simulink model "rx2"  (R2022b)
settings: Solver=FixedStepDiscrete  StartTime=0.0  StopTime=3.3E6  FixedStep=1  RelTol=1e-3  EnableMultiTasking=on
model workspace (MAT data in the model file):
  mwTaskManagerKernelLatency = 0
undefined symbols (not defined in the file or in its folder): Add, jsin, magnitude, rom_pilot_conj_tt, Shift
libraries: hdlsllib x3231, whdlutilities x525, simulink x260, whdlmod x112, whdledac x26, dsphdlmathfun2 x24, commchan3 x1
(part 5 of 59)

== system rx2/process divide/transport_block3/Subsystem8 ==
  data_in : Inport
  select_valid : Inport  Port=2  OutDataTypeStr=boolean
  Constant : Constant  Value=0  OutDataTypeStr=fixdt(1,16,14)
  Real-Imag to Complex : RealImagToComplex
  Switch : Switch  Criteria=u2 ~= 0  SaturateOnIntegerOverflow=off  InputSameDT=off
  ctrl_gen : Subsystem
  data_out : Outport
  ctrl_out : Outport  Port=2
  wires:
  Real-Imag to Complex/1 -> Switch/3
  data_in/1 -> Switch/1
  ctrl_gen/2(ctrl_out) -> ctrl_out/1
  ctrl_gen/1(data_out) -> data_out/1
  select_valid/1 -> Switch/2, ctrl_gen/2(valid_in)
  Constant/1 -> Real-Imag to Complex/1, Real-Imag to Complex/2
  Switch/1 -> ctrl_gen/1(data_in)

== system rx2/process divide/transport_block3/Subsystem9 ==
  data_in : Inport
  select_valid : Inport  Port=2  OutDataTypeStr=boolean
  Constant : Constant  Value=0  OutDataTypeStr=fixdt(1,16,14)
  Real-Imag to Complex : RealImagToComplex
  Switch : Switch  Criteria=u2 ~= 0  SaturateOnIntegerOverflow=off  InputSameDT=off
  ctrl_gen : Subsystem
  data_out : Outport
  ctrl_out : Outport  Port=2
  wires:
  Real-Imag to Complex/1 -> Switch/3
  data_in/1 -> Switch/1
  ctrl_gen/2(ctrl_out) -> ctrl_out/1
  ctrl_gen/1(data_out) -> data_out/1
  select_valid/1 -> Switch/2, ctrl_gen/2(valid_in)
  Constant/1 -> Real-Imag to Complex/1, Real-Imag to Complex/2
  Switch/1 -> ctrl_gen/1(data_in)

== system rx2/process divide/transport_block4/Subsystem1 ==
  data_in : Inport
  select_valid : Inport  Port=2  OutDataTypeStr=boolean
  Constant : Constant  Value=0  OutDataTypeStr=fixdt(1,16,14)
  Real-Imag to Complex : RealImagToComplex
  Switch : Switch  Criteria=u2 ~= 0  SaturateOnIntegerOverflow=off  InputSameDT=off
  ctrl_gen : Subsystem
  data_out : Outport
  ctrl_out : Outport  Port=2
  wires:
  Real-Imag to Complex/1 -> Switch/3
  data_in/1 -> Switch/1
  ctrl_gen/2(ctrl_out) -> ctrl_out/1
  ctrl_gen/1(data_out) -> data_out/1
  select_valid/1 -> Switch/2, ctrl_gen/2(valid_in)
  Constant/1 -> Real-Imag to Complex/1, Real-Imag to Complex/2
  Switch/1 -> ctrl_gen/1(data_in)

== system rx2/process divide/transport_block4/Subsystem10 ==
  data_in : Inport
  select_valid : Inport  Port=2  OutDataTypeStr=boolean
  Constant : Constant  Value=0  OutDataTypeStr=fixdt(1,16,14)
  Real-Imag to Complex : RealImagToComplex
  Switch : Switch  Criteria=u2 ~= 0  SaturateOnIntegerOverflow=off  InputSameDT=off
  ctrl_gen : Subsystem
  data_out : Outport
  ctrl_out : Outport  Port=2
  wires:
  Switch/1 -> ctrl_gen/1(data_in)
  Constant/1 -> Real-Imag to Complex/2, Real-Imag to Complex/1
  select_valid/1 -> ctrl_gen/2(valid_in), Switch/2
  ctrl_gen/1(data_out) -> data_out/1
  ctrl_gen/2(ctrl_out) -> ctrl_out/1
  data_in/1 -> Switch/1
  Real-Imag to Complex/1 -> Switch/3

== system rx2/process divide/transport_block4/Subsystem11 ==
  data_in : Inport
  select_valid : Inport  Port=2  OutDataTypeStr=boolean
  Constant : Constant  Value=0  OutDataTypeStr=fixdt(1,16,14)
  Real-Imag to Complex : RealImagToComplex
  Switch : Switch  Criteria=u2 ~= 0  SaturateOnIntegerOverflow=off  InputSameDT=off
  ctrl_gen : Subsystem
  data_out : Outport
  ctrl_out : Outport  Port=2
  wires:
  Switch/1 -> ctrl_gen/1(data_in)
  Constant/1 -> Real-Imag to Complex/2, Real-Imag to Complex/1
  select_valid/1 -> ctrl_gen/2(valid_in), Switch/2
  ctrl_gen/1(data_out) -> data_out/1
  ctrl_gen/2(ctrl_out) -> ctrl_out/1
  data_in/1 -> Switch/1
  Real-Imag to Complex/1 -> Switch/3

== system rx2/process divide/transport_block4/Subsystem12 ==
  data_in : Inport
  select_valid : Inport  Port=2  OutDataTypeStr=boolean
  Constant : Constant  Value=0  OutDataTypeStr=fixdt(1,16,14)
  Real-Imag to Complex : RealImagToComplex
  Switch : Switch  Criteria=u2 ~= 0  SaturateOnIntegerOverflow=off  InputSameDT=off
  ctrl_gen : Subsystem
  data_out : Outport
  ctrl_out : Outport  Port=2
  wires:
  Switch/1 -> ctrl_gen/1(data_in)
  Constant/1 -> Real-Imag to Complex/2, Real-Imag to Complex/1
  select_valid/1 -> ctrl_gen/2(valid_in), Switch/2
  ctrl_gen/1(data_out) -> data_out/1
  ctrl_gen/2(ctrl_out) -> ctrl_out/1
  data_in/1 -> Switch/1
  Real-Imag to Complex/1 -> Switch/3

== system rx2/process divide/transport_block4/Subsystem13 ==
  data_in : Inport
  select_valid : Inport  Port=2  OutDataTypeStr=boolean
  Constant : Constant  Value=0  OutDataTypeStr=fixdt(1,16,14)
  Real-Imag to Complex : RealImagToComplex
  Switch : Switch  Criteria=u2 ~= 0  SaturateOnIntegerOverflow=off  InputSameDT=off
  ctrl_gen : Subsystem
  data_out : Outport
  ctrl_out : Outport  Port=2
  wires:
  Switch/1 -> ctrl_gen/1(data_in)
  Constant/1 -> Real-Imag to Complex/2, Real-Imag to Complex/1
  select_valid/1 -> ctrl_gen/2(valid_in), Switch/2
  ctrl_gen/1(data_out) -> data_out/1
  ctrl_gen/2(ctrl_out) -> ctrl_out/1
  data_in/1 -> Switch/1
  Real-Imag to Complex/1 -> Switch/3

== system rx2/process divide/transport_block4/Subsystem14 ==
  data_in : Inport
  select_valid : Inport  Port=2  OutDataTypeStr=boolean
  Constant : Constant  Value=0  OutDataTypeStr=fixdt(1,16,14)
  Real-Imag to Complex : RealImagToComplex
  Switch : Switch  Criteria=u2 ~= 0  SaturateOnIntegerOverflow=off  InputSameDT=off
  ctrl_gen : Subsystem
  data_out : Outport
  ctrl_out : Outport  Port=2
  wires:
  Switch/1 -> ctrl_gen/1(data_in)
  Constant/1 -> Real-Imag to Complex/2, Real-Imag to Complex/1
  select_valid/1 -> ctrl_gen/2(valid_in), Switch/2
  ctrl_gen/1(data_out) -> data_out/1
  ctrl_gen/2(ctrl_out) -> ctrl_out/1
  data_in/1 -> Switch/1
  Real-Imag to Complex/1 -> Switch/3

== system rx2/process divide/transport_block4/Subsystem2 ==
  data_in : Inport
  select_valid : Inport  Port=2  OutDataTypeStr=boolean
  Constant : Constant  Value=0  OutDataTypeStr=fixdt(1,16,14)
  Real-Imag to Complex : RealImagToComplex
  Switch : Switch  Criteria=u2 ~= 0  SaturateOnIntegerOverflow=off  InputSameDT=off
  ctrl_gen : Subsystem
  data_out : Outport
  ctrl_out : Outport  Port=2
  wires:
  Switch/1 -> ctrl_gen/1(data_in)
  Constant/1 -> Real-Imag to Complex/2, Real-Imag to Complex/1
  select_valid/1 -> ctrl_gen/2(valid_in), Switch/2
  ctrl_gen/1(data_out) -> data_out/1
  ctrl_gen/2(ctrl_out) -> ctrl_out/1
  data_in/1 -> Switch/1
  Real-Imag to Complex/1 -> Switch/3

== system rx2/process divide/transport_block4/Subsystem3 ==
  data_in : Inport
  select_valid : Inport  Port=2  OutDataTypeStr=boolean
  Constant : Constant  Value=0  OutDataTypeStr=fixdt(1,16,14)
  Real-Imag to Complex : RealImagToComplex
  Switch : Switch  Criteria=u2 ~= 0  SaturateOnIntegerOverflow=off  InputSameDT=off
  ctrl_gen : Subsystem
  data_out : Outport
  ctrl_out : Outport  Port=2
  wires:
  Real-Imag to Complex/1 -> Switch/3
  data_in/1 -> Switch/1
  ctrl_gen/2(ctrl_out) -> ctrl_out/1
  ctrl_gen/1(data_out) -> data_out/1
  select_valid/1 -> Switch/2, ctrl_gen/2(valid_in)
  Constant/1 -> Real-Imag to Complex/1, Real-Imag to Complex/2
  Switch/1 -> ctrl_gen/1(data_in)

== system rx2/process divide/transport_block4/Subsystem4 ==
  data_in : Inport
  select_valid : Inport  Port=2  OutDataTypeStr=boolean
  Constant : Constant  Value=0  OutDataTypeStr=fixdt(1,16,14)
  Real-Imag to Complex : RealImagToComplex
  Switch : Switch  Criteria=u2 ~= 0  SaturateOnIntegerOverflow=off  InputSameDT=off
  ctrl_gen : Subsystem
  data_out : Outport
  ctrl_out : Outport  Port=2
  wires:
  Switch/1 -> ctrl_gen/1(data_in)
  Constant/1 -> Real-Imag to Complex/2, Real-Imag to Complex/1
  select_valid/1 -> ctrl_gen/2(valid_in), Switch/2
  ctrl_gen/1(data_out) -> data_out/1
  ctrl_gen/2(ctrl_out) -> ctrl_out/1
  data_in/1 -> Switch/1
  Real-Imag to Complex/1 -> Switch/3

== system rx2/process divide/transport_block4/Subsystem5 ==
  data_in : Inport
  select_valid : Inport  Port=2  OutDataTypeStr=boolean
  Constant : Constant  Value=0  OutDataTypeStr=fixdt(1,16,14)
  Real-Imag to Complex : RealImagToComplex
  Switch : Switch  Criteria=u2 ~= 0  SaturateOnIntegerOverflow=off  InputSameDT=off
  ctrl_gen : Subsystem
  data_out : Outport
  ctrl_out : Outport  Port=2
  wires:
  Switch/1 -> ctrl_gen/1(data_in)
  Constant/1 -> Real-Imag to Complex/2, Real-Imag to Complex/1
  select_valid/1 -> ctrl_gen/2(valid_in), Switch/2
  ctrl_gen/1(data_out) -> data_out/1
  ctrl_gen/2(ctrl_out) -> ctrl_out/1
  data_in/1 -> Switch/1
  Real-Imag to Complex/1 -> Switch/3

== system rx2/process divide/transport_block4/Subsystem6 ==
  data_in : Inport
  select_valid : Inport  Port=2  OutDataTypeStr=boolean
  Constant : Constant  Value=0  OutDataTypeStr=fixdt(1,16,14)
  Real-Imag to Complex : RealImagToComplex
  Switch : Switch  Criteria=u2 ~= 0  SaturateOnIntegerOverflow=off  InputSameDT=off
  ctrl_gen : Subsystem
  data_out : Outport
  ctrl_out : Outport  Port=2
  wires:
  Switch/1 -> ctrl_gen/1(data_in)
  Constant/1 -> Real-Imag to Complex/2, Real-Imag to Complex/1
  select_valid/1 -> ctrl_gen/2(valid_in), Switch/2
  ctrl_gen/1(data_out) -> data_out/1
  ctrl_gen/2(ctrl_out) -> ctrl_out/1
  data_in/1 -> Switch/1
  Real-Imag to Complex/1 -> Switch/3

== system rx2/process divide/transport_block4/Subsystem7 ==
  data_in : Inport
  select_valid : Inport  Port=2  OutDataTypeStr=boolean
  Constant : Constant  Value=0  OutDataTypeStr=fixdt(1,16,14)
  Real-Imag to Complex : RealImagToComplex
  Switch : Switch  Criteria=u2 ~= 0  SaturateOnIntegerOverflow=off  InputSameDT=off
  ctrl_gen : Subsystem
  data_out : Outport
  ctrl_out : Outport  Port=2
  wires:
  Switch/1 -> ctrl_gen/1(data_in)
  Constant/1 -> Real-Imag to Complex/2, Real-Imag to Complex/1
  select_valid/1 -> ctrl_gen/2(valid_in), Switch/2
  ctrl_gen/1(data_out) -> data_out/1
  ctrl_gen/2(ctrl_out) -> ctrl_out/1
  data_in/1 -> Switch/1
  Real-Imag to Complex/1 -> Switch/3

== system rx2/process divide/transport_block4/Subsystem8 ==
  data_in : Inport
  select_valid : Inport  Port=2  OutDataTypeStr=boolean
  Constant : Constant  Value=0  OutDataTypeStr=fixdt(1,16,14)
  Real-Imag to Complex : RealImagToComplex
  Switch : Switch  Criteria=u2 ~= 0  SaturateOnIntegerOverflow=off  InputSameDT=off
  ctrl_gen : Subsystem
  data_out : Outport
  ctrl_out : Outport  Port=2
  wires:
  Switch/1 -> ctrl_gen/1(data_in)
  Constant/1 -> Real-Imag to Complex/2, Real-Imag to Complex/1
  select_valid/1 -> ctrl_gen/2(valid_in), Switch/2
  ctrl_gen/1(data_out) -> data_out/1
  ctrl_gen/2(ctrl_out) -> ctrl_out/1
  data_in/1 -> Switch/1
  Real-Imag to Complex/1 -> Switch/3

== system rx2/process divide/transport_block4/Subsystem9 ==
  data_in : Inport
  select_valid : Inport  Port=2  OutDataTypeStr=boolean
  Constant : Constant  Value=0  OutDataTypeStr=fixdt(1,16,14)
  Real-Imag to Complex : RealImagToComplex
  Switch : Switch  Criteria=u2 ~= 0  SaturateOnIntegerOverflow=off  InputSameDT=off
  ctrl_gen : Subsystem
  data_out : Outport
  ctrl_out : Outport  Port=2
  wires:
  Switch/1 -> ctrl_gen/1(data_in)
  Constant/1 -> Real-Imag to Complex/2, Real-Imag to Complex/1
  select_valid/1 -> ctrl_gen/2(valid_in), Switch/2
  ctrl_gen/1(data_out) -> data_out/1
  ctrl_gen/2(ctrl_out) -> ctrl_out/1
  data_in/1 -> Switch/1
  Real-Imag to Complex/1 -> Switch/3

== system rx2/process divide/transport_block5/Subsystem1 ==
  data_in : Inport
  select_valid : Inport  Port=2  OutDataTypeStr=boolean
  Constant : Constant  Value=0  OutDataTypeStr=fixdt(1,16,14)
  Real-Imag to Complex : RealImagToComplex
  Switch : Switch  Criteria=u2 ~= 0  SaturateOnIntegerOverflow=off  InputSameDT=off
  ctrl_gen : Subsystem
  data_out : Outport
  ctrl_out : Outport  Port=2
  wires:
  Switch/1 -> ctrl_gen/1(data_in)
  Constant/1 -> Real-Imag to Complex/2, Real-Imag to Complex/1
  select_valid/1 -> ctrl_gen/2(valid_in), Switch/2
  ctrl_gen/1(data_out) -> data_out/1
  ctrl_gen/2(ctrl_out) -> ctrl_out/1
  data_in/1 -> Switch/1
  Real-Imag to Complex/1 -> Switch/3

== system rx2/process divide/transport_block5/Subsystem10 ==
  data_in : Inport
  select_valid : Inport  Port=2  OutDataTypeStr=boolean
  Constant : Constant  Value=0  OutDataTypeStr=fixdt(1,16,14)
  Real-Imag to Complex : RealImagToComplex
  Switch : Switch  Criteria=u2 ~= 0  SaturateOnIntegerOverflow=off  InputSameDT=off
  ctrl_gen : Subsystem
  data_out : Outport
  ctrl_out : Outport  Port=2
  wires:
  Real-Imag to Complex/1 -> Switch/3
  data_in/1 -> Switch/1
  ctrl_gen/2(ctrl_out) -> ctrl_out/1
  ctrl_gen/1(data_out) -> data_out/1
  select_valid/1 -> Switch/2, ctrl_gen/2(valid_in)
  Constant/1 -> Real-Imag to Complex/1, Real-Imag to Complex/2
  Switch/1 -> ctrl_gen/1(data_in)

== system rx2/process divide/transport_block5/Subsystem11 ==
  data_in : Inport
  select_valid : Inport  Port=2  OutDataTypeStr=boolean
  Constant : Constant  Value=0  OutDataTypeStr=fixdt(1,16,14)
  Real-Imag to Complex : RealImagToComplex
  Switch : Switch  Criteria=u2 ~= 0  SaturateOnIntegerOverflow=off  InputSameDT=off
  ctrl_gen : Subsystem
  data_out : Outport
  ctrl_out : Outport  Port=2
  wires:
  Real-Imag to Complex/1 -> Switch/3
  data_in/1 -> Switch/1
  ctrl_gen/2(ctrl_out) -> ctrl_out/1
  ctrl_gen/1(data_out) -> data_out/1
  select_valid/1 -> Switch/2, ctrl_gen/2(valid_in)
  Constant/1 -> Real-Imag to Complex/1, Real-Imag to Complex/2
  Switch/1 -> ctrl_gen/1(data_in)

== system rx2/process divide/transport_block5/Subsystem12 ==
  data_in : Inport
  select_valid : Inport  Port=2  OutDataTypeStr=boolean
  Constant : Constant  Value=0  OutDataTypeStr=fixdt(1,16,14)
  Real-Imag to Complex : RealImagToComplex
  Switch : Switch  Criteria=u2 ~= 0  SaturateOnIntegerOverflow=off  InputSameDT=off
  ctrl_gen : Subsystem
  data_out : Outport
  ctrl_out : Outport  Port=2
  wires:
  Real-Imag to Complex/1 -> Switch/3
  data_in/1 -> Switch/1
  ctrl_gen/2(ctrl_out) -> ctrl_out/1
  ctrl_gen/1(data_out) -> data_out/1
  select_valid/1 -> Switch/2, ctrl_gen/2(valid_in)
  Constant/1 -> Real-Imag to Complex/1, Real-Imag to Complex/2
  Switch/1 -> ctrl_gen/1(data_in)

== system rx2/process divide/transport_block5/Subsystem13 ==
  data_in : Inport
  select_valid : Inport  Port=2  OutDataTypeStr=boolean
  Constant : Constant  Value=0  OutDataTypeStr=fixdt(1,16,14)
  Real-Imag to Complex : RealImagToComplex
  Switch : Switch  Criteria=u2 ~= 0  SaturateOnIntegerOverflow=off  InputSameDT=off
  ctrl_gen : Subsystem
  data_out : Outport
  ctrl_out : Outport  Port=2
  wires:
  Real-Imag to Complex/1 -> Switch/3
  data_in/1 -> Switch/1
  ctrl_gen/2(ctrl_out) -> ctrl_out/1
  ctrl_gen/1(data_out) -> data_out/1
  select_valid/1 -> Switch/2, ctrl_gen/2(valid_in)
  Constant/1 -> Real-Imag to Complex/1, Real-Imag to Complex/2
  Switch/1 -> ctrl_gen/1(data_in)

== system rx2/process divide/transport_block5/Subsystem14 ==
  data_in : Inport
  select_valid : Inport  Port=2  OutDataTypeStr=boolean
  Constant : Constant  Value=0  OutDataTypeStr=fixdt(1,16,14)
  Real-Imag to Complex : RealImagToComplex
  Switch : Switch  Criteria=u2 ~= 0  SaturateOnIntegerOverflow=off  InputSameDT=off
  ctrl_gen : Subsystem
  data_out : Outport
  ctrl_out : Outport  Port=2
  wires:
  Real-Imag to Complex/1 -> Switch/3
  data_in/1 -> Switch/1
  ctrl_gen/2(ctrl_out) -> ctrl_out/1
  ctrl_gen/1(data_out) -> data_out/1
  select_valid/1 -> Switch/2, ctrl_gen/2(valid_in)
  Constant/1 -> Real-Imag to Complex/1, Real-Imag to Complex/2
  Switch/1 -> ctrl_gen/1(data_in)

== system rx2/process divide/transport_block5/Subsystem2 ==
  data_in : Inport
  select_valid : Inport  Port=2  OutDataTypeStr=boolean
  Constant : Constant  Value=0  OutDataTypeStr=fixdt(1,16,14)
  Real-Imag to Complex : RealImagToComplex
  Switch : Switch  Criteria=u2 ~= 0  SaturateOnIntegerOverflow=off  InputSameDT=off
  ctrl_gen : Subsystem
  data_out : Outport
  ctrl_out : Outport  Port=2
  wires:
  Real-Imag to Complex/1 -> Switch/3
  data_in/1 -> Switch/1
  ctrl_gen/2(ctrl_out) -> ctrl_out/1
  ctrl_gen/1(data_out) -> data_out/1
  select_valid/1 -> Switch/2, ctrl_gen/2(valid_in)
  Constant/1 -> Real-Imag to Complex/1, Real-Imag to Complex/2
  Switch/1 -> ctrl_gen/1(data_in)

== system rx2/process divide/transport_block5/Subsystem3 ==
  data_in : Inport
  select_valid : Inport  Port=2  OutDataTypeStr=boolean
  Constant : Constant  Value=0  OutDataTypeStr=fixdt(1,16,14)
  Real-Imag to Complex : RealImagToComplex
  Switch : Switch  Criteria=u2 ~= 0  SaturateOnIntegerOverflow=off  InputSameDT=off
  ctrl_gen : Subsystem
  data_out : Outport
  ctrl_out : Outport  Port=2
  wires:
  Switch/1 -> ctrl_gen/1(data_in)
  Constant/1 -> Real-Imag to Complex/2, Real-Imag to Complex/1
  select_valid/1 -> ctrl_gen/2(valid_in), Switch/2
  ctrl_gen/1(data_out) -> data_out/1
  ctrl_gen/2(ctrl_out) -> ctrl_out/1
  data_in/1 -> Switch/1
  Real-Imag to Complex/1 -> Switch/3

== system rx2/process divide/transport_block5/Subsystem4 ==
  data_in : Inport
  select_valid : Inport  Port=2  OutDataTypeStr=boolean
  Constant : Constant  Value=0  OutDataTypeStr=fixdt(1,16,14)
  Real-Imag to Complex : RealImagToComplex
  Switch : Switch  Criteria=u2 ~= 0  SaturateOnIntegerOverflow=off  InputSameDT=off
  ctrl_gen : Subsystem
  data_out : Outport
  ctrl_out : Outport  Port=2
  wires:
  Real-Imag to Complex/1 -> Switch/3
  data_in/1 -> Switch/1
  ctrl_gen/2(ctrl_out) -> ctrl_out/1
  ctrl_gen/1(data_out) -> data_out/1
  select_valid/1 -> Switch/2, ctrl_gen/2(valid_in)
  Constant/1 -> Real-Imag to Complex/1, Real-Imag to Complex/2
  Switch/1 -> ctrl_gen/1(data_in)

== system rx2/process divide/transport_block5/Subsystem5 ==
  data_in : Inport
  select_valid : Inport  Port=2  OutDataTypeStr=boolean
  Constant : Constant  Value=0  OutDataTypeStr=fixdt(1,16,14)
  Real-Imag to Complex : RealImagToComplex
  Switch : Switch  Criteria=u2 ~= 0  SaturateOnIntegerOverflow=off  InputSameDT=off
  ctrl_gen : Subsystem
  data_out : Outport
  ctrl_out : Outport  Port=2
  wires:
  Real-Imag to Complex/1 -> Switch/3
  data_in/1 -> Switch/1
  ctrl_gen/2(ctrl_out) -> ctrl_out/1
  ctrl_gen/1(data_out) -> data_out/1
  select_valid/1 -> Switch/2, ctrl_gen/2(valid_in)
  Constant/1 -> Real-Imag to Complex/1, Real-Imag to Complex/2
  Switch/1 -> ctrl_gen/1(data_in)

== system rx2/process divide/transport_block5/Subsystem6 ==
  data_in : Inport
  select_valid : Inport  Port=2  OutDataTypeStr=boolean
  Constant : Constant  Value=0  OutDataTypeStr=fixdt(1,16,14)
  Real-Imag to Complex : RealImagToComplex
  Switch : Switch  Criteria=u2 ~= 0  SaturateOnIntegerOverflow=off  InputSameDT=off
  ctrl_gen : Subsystem
  data_out : Outport
  ctrl_out : Outport  Port=2
  wires:
  Real-Imag to Complex/1 -> Switch/3
  data_in/1 -> Switch/1
  ctrl_gen/2(ctrl_out) -> ctrl_out/1
  ctrl_gen/1(data_out) -> data_out/1
  select_valid/1 -> Switch/2, ctrl_gen/2(valid_in)
  Constant/1 -> Real-Imag to Complex/1, Real-Imag to Complex/2
  Switch/1 -> ctrl_gen/1(data_in)

== system rx2/process divide/transport_block5/Subsystem7 ==
  data_in : Inport
  select_valid : Inport  Port=2  OutDataTypeStr=boolean
  Constant : Constant  Value=0  OutDataTypeStr=fixdt(1,16,14)
  Real-Imag to Complex : RealImagToComplex
  Switch : Switch  Criteria=u2 ~= 0  SaturateOnIntegerOverflow=off  InputSameDT=off
  ctrl_gen : Subsystem
  data_out : Outport
  ctrl_out : Outport  Port=2
  wires:
  Real-Imag to Complex/1 -> Switch/3
  data_in/1 -> Switch/1
  ctrl_gen/2(ctrl_out) -> ctrl_out/1
  ctrl_gen/1(data_out) -> data_out/1
  select_valid/1 -> Switch/2, ctrl_gen/2(valid_in)
  Constant/1 -> Real-Imag to Complex/1, Real-Imag to Complex/2
  Switch/1 -> ctrl_gen/1(data_in)

== system rx2/process divide/transport_block5/Subsystem8 ==
  data_in : Inport
  select_valid : Inport  Port=2  OutDataTypeStr=boolean
  Constant : Constant  Value=0  OutDataTypeStr=fixdt(1,16,14)
  Real-Imag to Complex : RealImagToComplex
  Switch : Switch  Criteria=u2 ~= 0  SaturateOnIntegerOverflow=off  InputSameDT=off
  ctrl_gen : Subsystem
  data_out : Outport
  ctrl_out : Outport  Port=2
  wires:
  Real-Imag to Complex/1 -> Switch/3
  data_in/1 -> Switch/1
  ctrl_gen/2(ctrl_out) -> ctrl_out/1
  ctrl_gen/1(data_out) -> data_out/1
  select_valid/1 -> Switch/2, ctrl_gen/2(valid_in)
  Constant/1 -> Real-Imag to Complex/1, Real-Imag to Complex/2
  Switch/1 -> ctrl_gen/1(data_in)

== system rx2/process divide/transport_block5/Subsystem9 ==
  data_in : Inport
  select_valid : Inport  Port=2  OutDataTypeStr=boolean
  Constant : Constant  Value=0  OutDataTypeStr=fixdt(1,16,14)
  Real-Imag to Complex : RealImagToComplex
  Switch : Switch  Criteria=u2 ~= 0  SaturateOnIntegerOverflow=off  InputSameDT=off
  ctrl_gen : Subsystem
  data_out : Outport
  ctrl_out : Outport  Port=2
  wires:
  Real-Imag to Complex/1 -> Switch/3
  data_in/1 -> Switch/1
  ctrl_gen/2(ctrl_out) -> ctrl_out/1
  ctrl_gen/1(data_out) -> data_out/1
  select_valid/1 -> Switch/2, ctrl_gen/2(valid_in)
  Constant/1 -> Real-Imag to Complex/1, Real-Imag to Complex/2
  Switch/1 -> ctrl_gen/1(data_in)

== system rx2/process divide/transport_block6/Subsystem1 ==
  data_in : Inport
  select_valid : Inport  Port=2  OutDataTypeStr=boolean
  Constant : Constant  Value=0  OutDataTypeStr=fixdt(1,16,14)
  Real-Imag to Complex : RealImagToComplex
  Switch : Switch  Criteria=u2 ~= 0  SaturateOnIntegerOverflow=off  InputSameDT=off
  ctrl_gen : Subsystem
  data_out : Outport
  ctrl_out : Outport  Port=2
  wires:
  Real-Imag to Complex/1 -> Switch/3
  data_in/1 -> Switch/1
  ctrl_gen/2(ctrl_out) -> ctrl_out/1
  ctrl_gen/1(data_out) -> data_out/1
  select_valid/1 -> Switch/2, ctrl_gen/2(valid_in)
  Constant/1 -> Real-Imag to Complex/1, Real-Imag to Complex/2
  Switch/1 -> ctrl_gen/1(data_in)

== system rx2/process divide/transport_block6/Subsystem10 ==
  data_in : Inport
  select_valid : Inport  Port=2  OutDataTypeStr=boolean
  Constant : Constant  Value=0  OutDataTypeStr=fixdt(1,16,14)
  Real-Imag to Complex : RealImagToComplex
  Switch : Switch  Criteria=u2 ~= 0  SaturateOnIntegerOverflow=off  InputSameDT=off
  ctrl_gen : Subsystem
  data_out : Outport
  ctrl_out : Outport  Port=2
  wires:
  Switch/1 -> ctrl_gen/1(data_in)
  Constant/1 -> Real-Imag to Complex/2, Real-Imag to Complex/1
  select_valid/1 -> ctrl_gen/2(valid_in), Switch/2
  ctrl_gen/1(data_out) -> data_out/1
  ctrl_gen/2(ctrl_out) -> ctrl_out/1
  data_in/1 -> Switch/1
  Real-Imag to Complex/1 -> Switch/3

== system rx2/process divide/transport_block6/Subsystem11 ==
  data_in : Inport
  select_valid : Inport  Port=2  OutDataTypeStr=boolean
  Constant : Constant  Value=0  OutDataTypeStr=fixdt(1,16,14)
  Real-Imag to Complex : RealImagToComplex
  Switch : Switch  Criteria=u2 ~= 0  SaturateOnIntegerOverflow=off  InputSameDT=off
  ctrl_gen : Subsystem
  data_out : Outport
  ctrl_out : Outport  Port=2
  wires:
  Switch/1 -> ctrl_gen/1(data_in)
  Constant/1 -> Real-Imag to Complex/2, Real-Imag to Complex/1
  select_valid/1 -> ctrl_gen/2(valid_in), Switch/2
  ctrl_gen/1(data_out) -> data_out/1
  ctrl_gen/2(ctrl_out) -> ctrl_out/1
  data_in/1 -> Switch/1
  Real-Imag to Complex/1 -> Switch/3

== system rx2/process divide/transport_block6/Subsystem12 ==
  data_in : Inport
  select_valid : Inport  Port=2  OutDataTypeStr=boolean
  Constant : Constant  Value=0  OutDataTypeStr=fixdt(1,16,14)
  Real-Imag to Complex : RealImagToComplex
  Switch : Switch  Criteria=u2 ~= 0  SaturateOnIntegerOverflow=off  InputSameDT=off
  ctrl_gen : Subsystem
  data_out : Outport
  ctrl_out : Outport  Port=2
  wires:
  Switch/1 -> ctrl_gen/1(data_in)
  Constant/1 -> Real-Imag to Complex/2, Real-Imag to Complex/1
  select_valid/1 -> ctrl_gen/2(valid_in), Switch/2
  ctrl_gen/1(data_out) -> data_out/1
  ctrl_gen/2(ctrl_out) -> ctrl_out/1
  data_in/1 -> Switch/1
  Real-Imag to Complex/1 -> Switch/3

== system rx2/process divide/transport_block6/Subsystem13 ==
  data_in : Inport
  select_valid : Inport  Port=2  OutDataTypeStr=boolean
  Constant : Constant  Value=0  OutDataTypeStr=fixdt(1,16,14)
  Real-Imag to Complex : RealImagToComplex
  Switch : Switch  Criteria=u2 ~= 0  SaturateOnIntegerOverflow=off  InputSameDT=off
  ctrl_gen : Subsystem
  data_out : Outport
  ctrl_out : Outport  Port=2
  wires:
  Switch/1 -> ctrl_gen/1(data_in)
  Constant/1 -> Real-Imag to Complex/2, Real-Imag to Complex/1
  select_valid/1 -> ctrl_gen/2(valid_in), Switch/2
  ctrl_gen/1(data_out) -> data_out/1
  ctrl_gen/2(ctrl_out) -> ctrl_out/1
  data_in/1 -> Switch/1
  Real-Imag to Complex/1 -> Switch/3

== system rx2/process divide/transport_block6/Subsystem14 ==
  data_in : Inport
  select_valid : Inport  Port=2  OutDataTypeStr=boolean
  Constant : Constant  Value=0  OutDataTypeStr=fixdt(1,16,14)
  Real-Imag to Complex : RealImagToComplex
  Switch : Switch  Criteria=u2 ~= 0  SaturateOnIntegerOverflow=off  InputSameDT=off
  ctrl_gen : Subsystem
  data_out : Outport
  ctrl_out : Outport  Port=2
  wires:
  Switch/1 -> ctrl_gen/1(data_in)
  Constant/1 -> Real-Imag to Complex/2, Real-Imag to Complex/1
  select_valid/1 -> ctrl_gen/2(valid_in), Switch/2
  ctrl_gen/1(data_out) -> data_out/1
  ctrl_gen/2(ctrl_out) -> ctrl_out/1
  data_in/1 -> Switch/1
  Real-Imag to Complex/1 -> Switch/3

== system rx2/process divide/transport_block6/Subsystem2 ==
  data_in : Inport
  select_valid : Inport  Port=2  OutDataTypeStr=boolean
  Constant : Constant  Value=0  OutDataTypeStr=fixdt(1,16,14)
  Real-Imag to Complex : RealImagToComplex
  Switch : Switch  Criteria=u2 ~= 0  SaturateOnIntegerOverflow=off  InputSameDT=off
  ctrl_gen : Subsystem
  data_out : Outport
  ctrl_out : Outport  Port=2
  wires:
  Switch/1 -> ctrl_gen/1(data_in)
  Constant/1 -> Real-Imag to Complex/2, Real-Imag to Complex/1
  select_valid/1 -> ctrl_gen/2(valid_in), Switch/2
  ctrl_gen/1(data_out) -> data_out/1
  ctrl_gen/2(ctrl_out) -> ctrl_out/1
  data_in/1 -> Switch/1
  Real-Imag to Complex/1 -> Switch/3

== system rx2/process divide/transport_block6/Subsystem3 ==
  data_in : Inport
  select_valid : Inport  Port=2  OutDataTypeStr=boolean
  Constant : Constant  Value=0  OutDataTypeStr=fixdt(1,16,14)
  Real-Imag to Complex : RealImagToComplex
  Switch : Switch  Criteria=u2 ~= 0  SaturateOnIntegerOverflow=off  InputSameDT=off
  ctrl_gen : Subsystem
  data_out : Outport
  ctrl_out : Outport  Port=2
  wires:
  Real-Imag to Complex/1 -> Switch/3
  data_in/1 -> Switch/1
  ctrl_gen/2(ctrl_out) -> ctrl_out/1
  ctrl_gen/1(data_out) -> data_out/1
  select_valid/1 -> Switch/2, ctrl_gen/2(valid_in)
  Constant/1 -> Real-Imag to Complex/1, Real-Imag to Complex/2
  Switch/1 -> ctrl_gen/1(data_in)

== system rx2/process divide/transport_block6/Subsystem4 ==
  data_in : Inport
  select_valid : Inport  Port=2  OutDataTypeStr=boolean
  Constant : Constant  Value=0  OutDataTypeStr=fixdt(1,16,14)
  Real-Imag to Complex : RealImagToComplex
  Switch : Switch  Criteria=u2 ~= 0  SaturateOnIntegerOverflow=off  InputSameDT=off
  ctrl_gen : Subsystem
  data_out : Outport
  ctrl_out : Outport  Port=2
  wires:
  Switch/1 -> ctrl_gen/1(data_in)
  Constant/1 -> Real-Imag to Complex/2, Real-Imag to Complex/1
  select_valid/1 -> ctrl_gen/2(valid_in), Switch/2
  ctrl_gen/1(data_out) -> data_out/1
  ctrl_gen/2(ctrl_out) -> ctrl_out/1
  data_in/1 -> Switch/1
  Real-Imag to Complex/1 -> Switch/3

== system rx2/process divide/transport_block6/Subsystem5 ==
  data_in : Inport
  select_valid : Inport  Port=2  OutDataTypeStr=boolean
  Constant : Constant  Value=0  OutDataTypeStr=fixdt(1,16,14)
  Real-Imag to Complex : RealImagToComplex
  Switch : Switch  Criteria=u2 ~= 0  SaturateOnIntegerOverflow=off  InputSameDT=off
  ctrl_gen : Subsystem
  data_out : Outport
  ctrl_out : Outport  Port=2
  wires:
  Switch/1 -> ctrl_gen/1(data_in)
  Constant/1 -> Real-Imag to Complex/2, Real-Imag to Complex/1
  select_valid/1 -> ctrl_gen/2(valid_in), Switch/2
  ctrl_gen/1(data_out) -> data_out/1
  ctrl_gen/2(ctrl_out) -> ctrl_out/1
  data_in/1 -> Switch/1
  Real-Imag to Complex/1 -> Switch/3

== system rx2/process divide/transport_block6/Subsystem6 ==
  data_in : Inport
  select_valid : Inport  Port=2  OutDataTypeStr=boolean
  Constant : Constant  Value=0  OutDataTypeStr=fixdt(1,16,14)
  Real-Imag to Complex : RealImagToComplex
  Switch : Switch  Criteria=u2 ~= 0  SaturateOnIntegerOverflow=off  InputSameDT=off
  ctrl_gen : Subsystem
  data_out : Outport
  ctrl_out : Outport  Port=2
  wires:
  Switch/1 -> ctrl_gen/1(data_in)
  Constant/1 -> Real-Imag to Complex/2, Real-Imag to Complex/1
  select_valid/1 -> ctrl_gen/2(valid_in), Switch/2
  ctrl_gen/1(data_out) -> data_out/1
  ctrl_gen/2(ctrl_out) -> ctrl_out/1
  data_in/1 -> Switch/1
  Real-Imag to Complex/1 -> Switch/3

== system rx2/process divide/transport_block6/Subsystem7 ==
  data_in : Inport
  select_valid : Inport  Port=2  OutDataTypeStr=boolean
  Constant : Constant  Value=0  OutDataTypeStr=fixdt(1,16,14)
  Real-Imag to Complex : RealImagToComplex
  Switch : Switch  Criteria=u2 ~= 0  SaturateOnIntegerOverflow=off  InputSameDT=off
  ctrl_gen : Subsystem
  data_out : Outport
  ctrl_out : Outport  Port=2
  wires:
  Switch/1 -> ctrl_gen/1(data_in)
  Constant/1 -> Real-Imag to Complex/2, Real-Imag to Complex/1
  select_valid/1 -> ctrl_gen/2(valid_in), Switch/2
  ctrl_gen/1(data_out) -> data_out/1
  ctrl_gen/2(ctrl_out) -> ctrl_out/1
  data_in/1 -> Switch/1
  Real-Imag to Complex/1 -> Switch/3

== system rx2/process divide/transport_block6/Subsystem8 ==
  data_in : Inport
  select_valid : Inport  Port=2  OutDataTypeStr=boolean
  Constant : Constant  Value=0  OutDataTypeStr=fixdt(1,16,14)
  Real-Imag to Complex : RealImagToComplex
  Switch : Switch  Criteria=u2 ~= 0  SaturateOnIntegerOverflow=off  InputSameDT=off
  ctrl_gen : Subsystem
  data_out : Outport
  ctrl_out : Outport  Port=2
  wires:
  Switch/1 -> ctrl_gen/1(data_in)
  Constant/1 -> Real-Imag to Complex/2, Real-Imag to Complex/1
  select_valid/1 -> ctrl_gen/2(valid_in), Switch/2
  ctrl_gen/1(data_out) -> data_out/1
  ctrl_gen/2(ctrl_out) -> ctrl_out/1
  data_in/1 -> Switch/1
  Real-Imag to Complex/1 -> Switch/3

== system rx2/process divide/transport_block6/Subsystem9 ==
  data_in : Inport
  select_valid : Inport  Port=2  OutDataTypeStr=boolean
  Constant : Constant  Value=0  OutDataTypeStr=fixdt(1,16,14)
  Real-Imag to Complex : RealImagToComplex
  Switch : Switch  Criteria=u2 ~= 0  SaturateOnIntegerOverflow=off  InputSameDT=off
  ctrl_gen : Subsystem
  data_out : Outport
  ctrl_out : Outport  Port=2
  wires:
  Switch/1 -> ctrl_gen/1(data_in)
  Constant/1 -> Real-Imag to Complex/2, Real-Imag to Complex/1
  select_valid/1 -> ctrl_gen/2(valid_in), Switch/2
  ctrl_gen/1(data_out) -> data_out/1
  ctrl_gen/2(ctrl_out) -> ctrl_out/1
  data_in/1 -> Switch/1
  Real-Imag to Complex/1 -> Switch/3

== system rx2/process divide/transport_block7/Subsystem1 ==
  data_in : Inport
  select_valid : Inport  Port=2  OutDataTypeStr=boolean
  Constant : Constant  Value=0  OutDataTypeStr=fixdt(1,16,14)
  Real-Imag to Complex : RealImagToComplex
  Switch : Switch  Criteria=u2 ~= 0  SaturateOnIntegerOverflow=off  InputSameDT=off
  ctrl_gen : Subsystem
  data_out : Outport
  ctrl_out : Outport  Port=2
  wires:
  Switch/1 -> ctrl_gen/1(data_in)
  Constant/1 -> Real-Imag to Complex/2, Real-Imag to Complex/1
  select_valid/1 -> ctrl_gen/2(valid_in), Switch/2
  ctrl_gen/1(data_out) -> data_out/1
  ctrl_gen/2(ctrl_out) -> ctrl_out/1
  data_in/1 -> Switch/1
  Real-Imag to Complex/1 -> Switch/3

== system rx2/process divide/transport_block7/Subsystem10 ==
  data_in : Inport
  select_valid : Inport  Port=2  OutDataTypeStr=boolean
  Constant : Constant  Value=0  OutDataTypeStr=fixdt(1,16,14)
  Real-Imag to Complex : RealImagToComplex
  Switch : Switch  Criteria=u2 ~= 0  SaturateOnIntegerOverflow=off  InputSameDT=off
  ctrl_gen : Subsystem
  data_out : Outport
  ctrl_out : Outport  Port=2
  wires:
  Real-Imag to Complex/1 -> Switch/3
  data_in/1 -> Switch/1
  ctrl_gen/2(ctrl_out) -> ctrl_out/1
  ctrl_gen/1(data_out) -> data_out/1
  select_valid/1 -> Switch/2, ctrl_gen/2(valid_in)
  Constant/1 -> Real-Imag to Complex/1, Real-Imag to Complex/2
  Switch/1 -> ctrl_gen/1(data_in)

== system rx2/process divide/transport_block7/Subsystem11 ==
  data_in : Inport
  select_valid : Inport  Port=2  OutDataTypeStr=boolean
  Constant : Constant  Value=0  OutDataTypeStr=fixdt(1,16,14)
  Real-Imag to Complex : RealImagToComplex
  Switch : Switch  Criteria=u2 ~= 0  SaturateOnIntegerOverflow=off  InputSameDT=off
  ctrl_gen : Subsystem
  data_out : Outport
  ctrl_out : Outport  Port=2
  wires:
  Real-Imag to Complex/1 -> Switch/3
  data_in/1 -> Switch/1
  ctrl_gen/2(ctrl_out) -> ctrl_out/1
  ctrl_gen/1(data_out) -> data_out/1
  select_valid/1 -> Switch/2, ctrl_gen/2(valid_in)
  Constant/1 -> Real-Imag to Complex/1, Real-Imag to Complex/2
  Switch/1 -> ctrl_gen/1(data_in)

== system rx2/process divide/transport_block7/Subsystem12 ==
  data_in : Inport
  select_valid : Inport  Port=2  OutDataTypeStr=boolean
  Constant : Constant  Value=0  OutDataTypeStr=fixdt(1,16,14)
  Real-Imag to Complex : RealImagToComplex
  Switch : Switch  Criteria=u2 ~= 0  SaturateOnIntegerOverflow=off  InputSameDT=off
  ctrl_gen : Subsystem
  data_out : Outport
  ctrl_out : Outport  Port=2
  wires:
  Real-Imag to Complex/1 -> Switch/3
  data_in/1 -> Switch/1
  ctrl_gen/2(ctrl_out) -> ctrl_out/1
  ctrl_gen/1(data_out) -> data_out/1
  select_valid/1 -> Switch/2, ctrl_gen/2(valid_in)
  Constant/1 -> Real-Imag to Complex/1, Real-Imag to Complex/2
  Switch/1 -> ctrl_gen/1(data_in)

== system rx2/process divide/transport_block7/Subsystem13 ==
  data_in : Inport
  select_valid : Inport  Port=2  OutDataTypeStr=boolean
  Constant : Constant  Value=0  OutDataTypeStr=fixdt(1,16,14)
  Real-Imag to Complex : RealImagToComplex
  Switch : Switch  Criteria=u2 ~= 0  SaturateOnIntegerOverflow=off  InputSameDT=off
  ctrl_gen : Subsystem
  data_out : Outport
  ctrl_out : Outport  Port=2
  wires:
  Real-Imag to Complex/1 -> Switch/3
  data_in/1 -> Switch/1
  ctrl_gen/2(ctrl_out) -> ctrl_out/1
  ctrl_gen/1(data_out) -> data_out/1
  select_valid/1 -> Switch/2, ctrl_gen/2(valid_in)
  Constant/1 -> Real-Imag to Complex/1, Real-Imag to Complex/2
  Switch/1 -> ctrl_gen/1(data_in)

== system rx2/process divide/transport_block7/Subsystem14 ==
  data_in : Inport
  select_valid : Inport  Port=2  OutDataTypeStr=boolean
  Constant : Constant  Value=0  OutDataTypeStr=fixdt(1,16,14)
  Real-Imag to Complex : RealImagToComplex
  Switch : Switch  Criteria=u2 ~= 0  SaturateOnIntegerOverflow=off  InputSameDT=off
  ctrl_gen : Subsystem
  data_out : Outport
  ctrl_out : Outport  Port=2
  wires:
  Real-Imag to Complex/1 -> Switch/3
  data_in/1 -> Switch/1
  ctrl_gen/2(ctrl_out) -> ctrl_out/1
  ctrl_gen/1(data_out) -> data_out/1
  select_valid/1 -> Switch/2, ctrl_gen/2(valid_in)
  Constant/1 -> Real-Imag to Complex/1, Real-Imag to Complex/2
  Switch/1 -> ctrl_gen/1(data_in)

== system rx2/process divide/transport_block7/Subsystem2 ==
  data_in : Inport
  select_valid : Inport  Port=2  OutDataTypeStr=boolean
  Constant : Constant  Value=0  OutDataTypeStr=fixdt(1,16,14)
  Real-Imag to Complex : RealImagToComplex
  Switch : Switch  Criteria=u2 ~= 0  SaturateOnIntegerOverflow=off  InputSameDT=off
  ctrl_gen : Subsystem
  data_out : Outport
  ctrl_out : Outport  Port=2
  wires:
  Real-Imag to Complex/1 -> Switch/3
  data_in/1 -> Switch/1
  ctrl_gen/2(ctrl_out) -> ctrl_out/1
  ctrl_gen/1(data_out) -> data_out/1
  select_valid/1 -> Switch/2, ctrl_gen/2(valid_in)
  Constant/1 -> Real-Imag to Complex/1, Real-Imag to Complex/2
  Switch/1 -> ctrl_gen/1(data_in)

== system rx2/process divide/transport_block7/Subsystem3 ==
  data_in : Inport
  select_valid : Inport  Port=2  OutDataTypeStr=boolean
  Constant : Constant  Value=0  OutDataTypeStr=fixdt(1,16,14)
  Real-Imag to Complex : RealImagToComplex
  Switch : Switch  Criteria=u2 ~= 0  SaturateOnIntegerOverflow=off  InputSameDT=off
  ctrl_gen : Subsystem
  data_out : Outport
  ctrl_out : Outport  Port=2
  wires:
  Switch/1 -> ctrl_gen/1(data_in)
  Constant/1 -> Real-Imag to Complex/2, Real-Imag to Complex/1
  select_valid/1 -> ctrl_gen/2(valid_in), Switch/2
  ctrl_gen/1(data_out) -> data_out/1
  ctrl_gen/2(ctrl_out) -> ctrl_out/1
  data_in/1 -> Switch/1
  Real-Imag to Complex/1 -> Switch/3

== system rx2/process divide/transport_block7/Subsystem4 ==
  data_in : Inport
  select_valid : Inport  Port=2  OutDataTypeStr=boolean
  Constant : Constant  Value=0  OutDataTypeStr=fixdt(1,16,14)
  Real-Imag to Complex : RealImagToComplex
  Switch : Switch  Criteria=u2 ~= 0  SaturateOnIntegerOverflow=off  InputSameDT=off
  ctrl_gen : Subsystem
  data_out : Outport
  ctrl_out : Outport  Port=2
  wires:
  Real-Imag to Complex/1 -> Switch/3
  data_in/1 -> Switch/1
  ctrl_gen/2(ctrl_out) -> ctrl_out/1
  ctrl_gen/1(data_out) -> data_out/1
  select_valid/1 -> Switch/2, ctrl_gen/2(valid_in)
  Constant/1 -> Real-Imag to Complex/1, Real-Imag to Complex/2
  Switch/1 -> ctrl_gen/1(data_in)

== system rx2/process divide/transport_block7/Subsystem5 ==
  data_in : Inport
  select_valid : Inport  Port=2  OutDataTypeStr=boolean
  Constant : Constant  Value=0  OutDataTypeStr=fixdt(1,16,14)
  Real-Imag to Complex : RealImagToComplex
  Switch : Switch  Criteria=u2 ~= 0  SaturateOnIntegerOverflow=off  InputSameDT=off
  ctrl_gen : Subsystem
  data_out : Outport
  ctrl_out : Outport  Port=2
  wires:
  Real-Imag to Complex/1 -> Switch/3
  data_in/1 -> Switch/1
  ctrl_gen/2(ctrl_out) -> ctrl_out/1
  ctrl_gen/1(data_out) -> data_out/1
  select_valid/1 -> Switch/2, ctrl_gen/2(valid_in)
  Constant/1 -> Real-Imag to Complex/1, Real-Imag to Complex/2
  Switch/1 -> ctrl_gen/1(data_in)

== system rx2/process divide/transport_block7/Subsystem6 ==
  data_in : Inport
  select_valid : Inport  Port=2  OutDataTypeStr=boolean
  Constant : Constant  Value=0  OutDataTypeStr=fixdt(1,16,14)
  Real-Imag to Complex : RealImagToComplex
  Switch : Switch  Criteria=u2 ~= 0  SaturateOnIntegerOverflow=off  InputSameDT=off
  ctrl_gen : Subsystem
  data_out : Outport
  ctrl_out : Outport  Port=2
  wires:
  Real-Imag to Complex/1 -> Switch/3
  data_in/1 -> Switch/1
  ctrl_gen/2(ctrl_out) -> ctrl_out/1
  ctrl_gen/1(data_out) -> data_out/1
  select_valid/1 -> Switch/2, ctrl_gen/2(valid_in)
  Constant/1 -> Real-Imag to Complex/1, Real-Imag to Complex/2
  Switch/1 -> ctrl_gen/1(data_in)

== system rx2/process divide/transport_block7/Subsystem7 ==
  data_in : Inport
  select_valid : Inport  Port=2  OutDataTypeStr=boolean
  Constant : Constant  Value=0  OutDataTypeStr=fixdt(1,16,14)
  Real-Imag to Complex : RealImagToComplex
  Switch : Switch  Criteria=u2 ~= 0  SaturateOnIntegerOverflow=off  InputSameDT=off
  ctrl_gen : Subsystem
  data_out : Outport
  ctrl_out : Outport  Port=2
  wires:
  Real-Imag to Complex/1 -> Switch/3
  data_in/1 -> Switch/1
  ctrl_gen/2(ctrl_out) -> ctrl_out/1
  ctrl_gen/1(data_out) -> data_out/1
  select_valid/1 -> Switch/2, ctrl_gen/2(valid_in)
  Constant/1 -> Real-Imag to Complex/1, Real-Imag to Complex/2
  Switch/1 -> ctrl_gen/1(data_in)

== system rx2/process divide/transport_block7/Subsystem8 ==
  data_in : Inport
  select_valid : Inport  Port=2  OutDataTypeStr=boolean
  Constant : Constant  Value=0  OutDataTypeStr=fixdt(1,16,14)
  Real-Imag to Complex : RealImagToComplex
  Switch : Switch  Criteria=u2 ~= 0  SaturateOnIntegerOverflow=off  InputSameDT=off
  ctrl_gen : Subsystem
  data_out : Outport
  ctrl_out : Outport  Port=2
  wires:
  Real-Imag to Complex/1 -> Switch/3
  data_in/1 -> Switch/1
  ctrl_gen/2(ctrl_out) -> ctrl_out/1
  ctrl_gen/1(data_out) -> data_out/1
  select_valid/1 -> Switch/2, ctrl_gen/2(valid_in)
  Constant/1 -> Real-Imag to Complex/1, Real-Imag to Complex/2
  Switch/1 -> ctrl_gen/1(data_in)

== system rx2/process divide/transport_block7/Subsystem9 ==
  data_in : Inport
  select_valid : Inport  Port=2  OutDataTypeStr=boolean
  Constant : Constant  Value=0  OutDataTypeStr=fixdt(1,16,14)
  Real-Imag to Complex : RealImagToComplex
  Switch : Switch  Criteria=u2 ~= 0  SaturateOnIntegerOverflow=off  InputSameDT=off
  ctrl_gen : Subsystem
  data_out : Outport
  ctrl_out : Outport  Port=2
  wires:
  Real-Imag to Complex/1 -> Switch/3
  data_in/1 -> Switch/1
  ctrl_gen/2(ctrl_out) -> ctrl_out/1
  ctrl_gen/1(data_out) -> data_out/1
  select_valid/1 -> Switch/2, ctrl_gen/2(valid_in)
  Constant/1 -> Real-Imag to Complex/1, Real-Imag to Complex/2
  Switch/1 -> ctrl_gen/1(data_in)

== system rx2/process divide/transport_block8/Subsystem1 ==
  data_in : Inport
  select_valid : Inport  Port=2  OutDataTypeStr=boolean
  Constant : Constant  Value=0  OutDataTypeStr=fixdt(1,16,14)
  Real-Imag to Complex : RealImagToComplex
  Switch : Switch  Criteria=u2 ~= 0  SaturateOnIntegerOverflow=off  InputSameDT=off
  ctrl_gen : Subsystem
  data_out : Outport
  ctrl_out : Outport  Port=2
  wires:
  Real-Imag to Complex/1 -> Switch/3
  data_in/1 -> Switch/1
  ctrl_gen/2(ctrl_out) -> ctrl_out/1
  ctrl_gen/1(data_out) -> data_out/1
  select_valid/1 -> Switch/2, ctrl_gen/2(valid_in)
  Constant/1 -> Real-Imag to Complex/1, Real-Imag to Complex/2
  Switch/1 -> ctrl_gen/1(data_in)

== system rx2/process divide/transport_block8/Subsystem10 ==
  data_in : Inport
  select_valid : Inport  Port=2  OutDataTypeStr=boolean
  Constant : Constant  Value=0  OutDataTypeStr=fixdt(1,16,14)
  Real-Imag to Complex : RealImagToComplex
  Switch : Switch  Criteria=u2 ~= 0  SaturateOnIntegerOverflow=off  InputSameDT=off
  ctrl_gen : Subsystem
  data_out : Outport
  ctrl_out : Outport  Port=2
  wires:
  Switch/1 -> ctrl_gen/1(data_in)
  Constant/1 -> Real-Imag to Complex/2, Real-Imag to Complex/1
  select_valid/1 -> ctrl_gen/2(valid_in), Switch/2
  ctrl_gen/1(data_out) -> data_out/1
  ctrl_gen/2(ctrl_out) -> ctrl_out/1
  data_in/1 -> Switch/1
  Real-Imag to Complex/1 -> Switch/3

== system rx2/process divide/transport_block8/Subsystem11 ==
  data_in : Inport
  select_valid : Inport  Port=2  OutDataTypeStr=boolean
  Constant : Constant  Value=0  OutDataTypeStr=fixdt(1,16,14)
  Real-Imag to Complex : RealImagToComplex
  Switch : Switch  Criteria=u2 ~= 0  SaturateOnIntegerOverflow=off  InputSameDT=off
  ctrl_gen : Subsystem
  data_out : Outport
  ctrl_out : Outport  Port=2
  wires:
  Switch/1 -> ctrl_gen/1(data_in)
  Constant/1 -> Real-Imag to Complex/2, Real-Imag to Complex/1
  select_valid/1 -> ctrl_gen/2(valid_in), Switch/2
  ctrl_gen/1(data_out) -> data_out/1
  ctrl_gen/2(ctrl_out) -> ctrl_out/1
  data_in/1 -> Switch/1
  Real-Imag to Complex/1 -> Switch/3

== system rx2/process divide/transport_block8/Subsystem12 ==
  data_in : Inport
  select_valid : Inport  Port=2  OutDataTypeStr=boolean
  Constant : Constant  Value=0  OutDataTypeStr=fixdt(1,16,14)
  Real-Imag to Complex : RealImagToComplex
  Switch : Switch  Criteria=u2 ~= 0  SaturateOnIntegerOverflow=off  InputSameDT=off
  ctrl_gen : Subsystem
  data_out : Outport
  ctrl_out : Outport  Port=2
  wires:
  Switch/1 -> ctrl_gen/1(data_in)
  Constant/1 -> Real-Imag to Complex/2, Real-Imag to Complex/1
  select_valid/1 -> ctrl_gen/2(valid_in), Switch/2
  ctrl_gen/1(data_out) -> data_out/1
  ctrl_gen/2(ctrl_out) -> ctrl_out/1
  data_in/1 -> Switch/1
  Real-Imag to Complex/1 -> Switch/3

== system rx2/process divide/transport_block8/Subsystem13 ==
  data_in : Inport
  select_valid : Inport  Port=2  OutDataTypeStr=boolean
  Constant : Constant  Value=0  OutDataTypeStr=fixdt(1,16,14)
  Real-Imag to Complex : RealImagToComplex
  Switch : Switch  Criteria=u2 ~= 0  SaturateOnIntegerOverflow=off  InputSameDT=off
  ctrl_gen : Subsystem
  data_out : Outport
  ctrl_out : Outport  Port=2
  wires:
  Switch/1 -> ctrl_gen/1(data_in)
  Constant/1 -> Real-Imag to Complex/2, Real-Imag to Complex/1
  select_valid/1 -> ctrl_gen/2(valid_in), Switch/2
  ctrl_gen/1(data_out) -> data_out/1
  ctrl_gen/2(ctrl_out) -> ctrl_out/1
  data_in/1 -> Switch/1
  Real-Imag to Complex/1 -> Switch/3

== system rx2/process divide/transport_block8/Subsystem14 ==
  data_in : Inport
  select_valid : Inport  Port=2  OutDataTypeStr=boolean
  Constant : Constant  Value=0  OutDataTypeStr=fixdt(1,16,14)
  Real-Imag to Complex : RealImagToComplex
  Switch : Switch  Criteria=u2 ~= 0  SaturateOnIntegerOverflow=off  InputSameDT=off
  ctrl_gen : Subsystem
  data_out : Outport
  ctrl_out : Outport  Port=2
  wires:
  Switch/1 -> ctrl_gen/1(data_in)
  Constant/1 -> Real-Imag to Complex/2, Real-Imag to Complex/1
  select_valid/1 -> ctrl_gen/2(valid_in), Switch/2
  ctrl_gen/1(data_out) -> data_out/1
  ctrl_gen/2(ctrl_out) -> ctrl_out/1
  data_in/1 -> Switch/1
  Real-Imag to Complex/1 -> Switch/3

== system rx2/process divide/transport_block8/Subsystem2 ==
  data_in : Inport
  select_valid : Inport  Port=2  OutDataTypeStr=boolean
  Constant : Constant  Value=0  OutDataTypeStr=fixdt(1,16,14)
  Real-Imag to Complex : RealImagToComplex
  Switch : Switch  Criteria=u2 ~= 0  SaturateOnIntegerOverflow=off  InputSameDT=off
  ctrl_gen : Subsystem
  data_out : Outport
  ctrl_out : Outport  Port=2
  wires:
  Switch/1 -> ctrl_gen/1(data_in)
  Constant/1 -> Real-Imag to Complex/2, Real-Imag to Complex/1
  select_valid/1 -> ctrl_gen/2(valid_in), Switch/2
  ctrl_gen/1(data_out) -> data_out/1
  ctrl_gen/2(ctrl_out) -> ctrl_out/1
  data_in/1 -> Switch/1
  Real-Imag to Complex/1 -> Switch/3

== system rx2/process divide/transport_block8/Subsystem3 ==
  data_in : Inport
  select_valid : Inport  Port=2  OutDataTypeStr=boolean
  Constant : Constant  Value=0  OutDataTypeStr=fixdt(1,16,14)
  Real-Imag to Complex : RealImagToComplex
  Switch : Switch  Criteria=u2 ~= 0  SaturateOnIntegerOverflow=off  InputSameDT=off
  ctrl_gen : Subsystem
  data_out : Outport
  ctrl_out : Outport  Port=2
  wires:
  Real-Imag to Complex/1 -> Switch/3
  data_in/1 -> Switch/1
  ctrl_gen/2(ctrl_out) -> ctrl_out/1
  ctrl_gen/1(data_out) -> data_out/1
  select_valid/1 -> Switch/2, ctrl_gen/2(valid_in)
  Constant/1 -> Real-Imag to Complex/1, Real-Imag to Complex/2
  Switch/1 -> ctrl_gen/1(data_in)

== system rx2/process divide/transport_block8/Subsystem4 ==
  data_in : Inport
  select_valid : Inport  Port=2  OutDataTypeStr=boolean
  Constant : Constant  Value=0  OutDataTypeStr=fixdt(1,16,14)
  Real-Imag to Complex : RealImagToComplex
  Switch : Switch  Criteria=u2 ~= 0  SaturateOnIntegerOverflow=off  InputSameDT=off
  ctrl_gen : Subsystem
  data_out : Outport
  ctrl_out : Outport  Port=2
  wires:
  Switch/1 -> ctrl_gen/1(data_in)
  Constant/1 -> Real-Imag to Complex/2, Real-Imag to Complex/1
  select_valid/1 -> ctrl_gen/2(valid_in), Switch/2
  ctrl_gen/1(data_out) -> data_out/1
  ctrl_gen/2(ctrl_out) -> ctrl_out/1
  data_in/1 -> Switch/1
  Real-Imag to Complex/1 -> Switch/3

== system rx2/process divide/transport_block8/Subsystem5 ==
  data_in : Inport
  select_valid : Inport  Port=2  OutDataTypeStr=boolean
  Constant : Constant  Value=0  OutDataTypeStr=fixdt(1,16,14)
  Real-Imag to Complex : RealImagToComplex
  Switch : Switch  Criteria=u2 ~= 0  SaturateOnIntegerOverflow=off  InputSameDT=off
  ctrl_gen : Subsystem
  data_out : Outport
  ctrl_out : Outport  Port=2
  wires:
  Switch/1 -> ctrl_gen/1(data_in)
  Constant/1 -> Real-Imag to Complex/2, Real-Imag to Complex/1
  select_valid/1 -> ctrl_gen/2(valid_in), Switch/2
  ctrl_gen/1(data_out) -> data_out/1
  ctrl_gen/2(ctrl_out) -> ctrl_out/1
  data_in/1 -> Switch/1
  Real-Imag to Complex/1 -> Switch/3

== system rx2/process divide/transport_block8/Subsystem6 ==
  data_in : Inport
  select_valid : Inport  Port=2  OutDataTypeStr=boolean
  Constant : Constant  Value=0  OutDataTypeStr=fixdt(1,16,14)
  Real-Imag to Complex : RealImagToComplex
  Switch : Switch  Criteria=u2 ~= 0  SaturateOnIntegerOverflow=off  InputSameDT=off
  ctrl_gen : Subsystem
  data_out : Outport
  ctrl_out : Outport  Port=2
  wires:
  Switch/1 -> ctrl_gen/1(data_in)
  Constant/1 -> Real-Imag to Complex/2, Real-Imag to Complex/1
  select_valid/1 -> ctrl_gen/2(valid_in), Switch/2
  ctrl_gen/1(data_out) -> data_out/1
  ctrl_gen/2(ctrl_out) -> ctrl_out/1
  data_in/1 -> Switch/1
  Real-Imag to Complex/1 -> Switch/3

== system rx2/process divide/transport_block8/Subsystem7 ==
  data_in : Inport
  select_valid : Inport  Port=2  OutDataTypeStr=boolean
  Constant : Constant  Value=0  OutDataTypeStr=fixdt(1,16,14)
  Real-Imag to Complex : RealImagToComplex
  Switch : Switch  Criteria=u2 ~= 0  SaturateOnIntegerOverflow=off  InputSameDT=off
  ctrl_gen : Subsystem
  data_out : Outport
  ctrl_out : Outport  Port=2
  wires:
  Switch/1 -> ctrl_gen/1(data_in)
  Constant/1 -> Real-Imag to Complex/2, Real-Imag to Complex/1
  select_valid/1 -> ctrl_gen/2(valid_in), Switch/2
  ctrl_gen/1(data_out) -> data_out/1
  ctrl_gen/2(ctrl_out) -> ctrl_out/1
  data_in/1 -> Switch/1
  Real-Imag to Complex/1 -> Switch/3

== system rx2/process divide/transport_block8/Subsystem8 ==
  data_in : Inport
  select_valid : Inport  Port=2  OutDataTypeStr=boolean
  Constant : Constant  Value=0  OutDataTypeStr=fixdt(1,16,14)
  Real-Imag to Complex : RealImagToComplex
  Switch : Switch  Criteria=u2 ~= 0  SaturateOnIntegerOverflow=off  InputSameDT=off
  ctrl_gen : Subsystem
  data_out : Outport
  ctrl_out : Outport  Port=2
  wires:
  Switch/1 -> ctrl_gen/1(data_in)
  Constant/1 -> Real-Imag to Complex/2, Real-Imag to Complex/1
  select_valid/1 -> ctrl_gen/2(valid_in), Switch/2
  ctrl_gen/1(data_out) -> data_out/1
  ctrl_gen/2(ctrl_out) -> ctrl_out/1
  data_in/1 -> Switch/1
  Real-Imag to Complex/1 -> Switch/3
